simulink model "model"  (R2018a)
settings: Solver=VariableStepAuto  StartTime=0.0  StopTime=0.01  MaxStep=1e-5  RelTol=1e-3
values from neighbouring files (symbols this model uses):
  Cp = 1/(4*pi^2*f^2*Lp)    (= 1.42505180932e-08)    [parametric_simulation.m]
  Cs = 1/(4*pi^2*f^2*Ls)    (= 1.63158105704e-08)    [parametric_simulation.m]
  fop = 156    [parametric_simulation.m]
  R_Load = 10    [parametric_simulation.m]
  Vin_peak = 127    [parametric_simulation.m]
libraries: powerlib x42
settings Model: Creator=user  LastModifiedBy=enes_

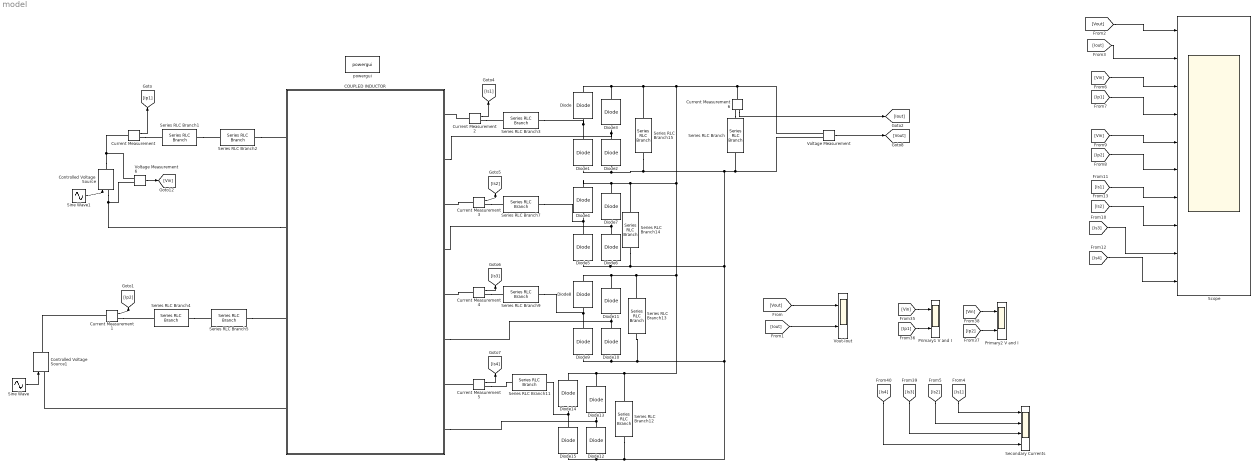
== system model ==
  COUPLED INDUCTOR : Subsystem
  Controlled Voltage Source : powerlib/Electrical Sources/Controlled Voltage Source  Initialize=on  Source_Type=AC  Amplitude=0  Phase=0  Frequency=0  Measurements=None
  Controlled Voltage Source1 : powerlib/Electrical Sources/Controlled Voltage Source  Initialize=on  Source_Type=AC  Amplitude=0  Phase=0  Frequency=0  Measurements=None
  Current Measurement{,1..6} (7 alike) : powerlib/Measurements/Current Measurement  PhasorSimulation=off  OutputType=Complex  PSBequivalent=0
  Diode{,1..15} (16 alike) : powerlib/Power Electronics/Diode  Ron=0.001  Lon=0  Vf=0.8  IC=0  UseSnubber=0  Rs=inf  Cs=250e-9  Measurements=off
  Primary1 V and I : Scope  NumInputPorts=2
  Primary2 V and I : Scope  NumInputPorts=2
  Scope : Scope  NumInputPorts=10
  Secondary Currents : Scope  NumInputPorts=4
  Series RLC Branch : powerlib/Elements/Series RLC Branch  LConnTagsString=__new0  RConnTagsString=__new0  BranchType=R  Resistance=R_Load  Inductance=1e-3  SetiL0=off  InitialCurrent=0  Capacitance=1e-6  Setx0=off  InitialVoltage=0  Measurements=None
  Series RLC Branch1 : powerlib/Elements/Series RLC Branch  LConnTagsString=__new0  RConnTagsString=__new0  BranchType=R  Resistance=0.01  Inductance=1e-3  SetiL0=off  InitialCurrent=0  Capacitance=1e-6  Setx0=off  InitialVoltage=0  Measurements=None
  Series RLC Branch{3,7,9,11} (4 alike) : powerlib/Elements/Series RLC Branch  LConnTagsString=__new0  RConnTagsString=__new0  BranchType=C  Resistance=0.01  Inductance=1e-3  SetiL0=off  InitialCurrent=0  Capacitance=Cs  Setx0=off  InitialVoltage=0  Measurements=None
  Series RLC Branch{12..15} (4 alike) : powerlib/Elements/Series RLC Branch  LConnTagsString=__new0  RConnTagsString=__new0  BranchType=C  Resistance=70  Inductance=1e-3  SetiL0=off  InitialCurrent=0  Capacitance=1e-6  Setx0=off  InitialVoltage=0  Measurements=None
  Series RLC Branch2 : powerlib/Elements/Series RLC Branch  LConnTagsString=__new0  RConnTagsString=__new0  BranchType=C  Resistance=0.01  Inductance=1e-3  SetiL0=off  InitialCurrent=0  Capacitance=Cp  Setx0=off  InitialVoltage=0  Measurements=None
  Series RLC Branch4 : powerlib/Elements/Series RLC Branch  LConnTagsString=__new0  RConnTagsString=__new0  BranchType=R  Resistance=0.01  Inductance=1e-3  SetiL0=off  InitialCurrent=0  Capacitance=1e-6  Setx0=off  InitialVoltage=0  Measurements=None
  Series RLC Branch5 : powerlib/Elements/Series RLC Branch  LConnTagsString=__new0  RConnTagsString=__new0  BranchType=C  Resistance=0.01  Inductance=1e-3  SetiL0=off  InitialCurrent=0  Capacitance=Cp  Setx0=off  InitialVoltage=0  Measurements=None
  Sine Wave : Sin  Amplitude=Vin_peak  Frequency=fop*1000*2*pi  SampleTime=0
  Sine Wave1 : Sin  Amplitude=Vin_peak  Frequency=fop*1000*2*pi  SampleTime=0
  Voltage Measurement : powerlib/Measurements/Voltage Measurement  PhasorSimulation=off  OutputType=Complex  PSBequivalent=0
  Voltage Measurement6 : powerlib/Measurements/Voltage Measurement  PhasorSimulation=off  OutputType=Complex  PSBequivalent=0
  Vout-Iout : Scope  NumInputPorts=2
  powergui : powerlib/powergui  Priority=1  SimulationMode=Continuous  SampleTime=50e-6  frequency=60  Iterations=50  frequencyindice=0  Pbase=100e6  ErrMax=1e-4  UnitsV=kV  UnitsW=MW  buscounter=0  FunctionMessages=off  echomessages=off  EnableUseOfTLC=off  CurrentSourceSwitches=off  DisableSnubberDevices=off  DisableRonSwitches=off  DisableVfSwitches=off  DisplayEquations=off  SolverType=Tustin/Backward Euler (TBE)  Interpol=off  ExternalGateDelay=off  methode=off  Ts=100  x0status=blocks  SPID=on  SwTol=0  HookPort=off  RestoreLinks=warning  ResistiveCurrentMeasurement=off  Frange=[0:2:500]  Ylog=off  Xlog=on  ShowGrid=off  save=off  variable=ZData  structure=0  ZoomFFT=off  StartTime=0.0  cycles=1  DisplayStyle=1  fundamental=60  FreqAxis=off  MaxFrequency=1000  frequencyindicesteady=1  RmsSteady=1  display=off
  wires:
  [Ip1] -> Primary1 V and I/2
  [Vin] -> Primary1 V and I/1
  [Vin] -> Primary2 V and I/1
  Current Measurement/1 -> [Ip1]
  Current Measurement4/1 -> [Is3]
  Current Measurement1/1 -> [Ip2]
  [Vout] -> Vout-Iout/1
  Sine Wave1/1 -> Controlled Voltage Source/1
  Current Measurement3/1 -> [Is2]
  Voltage Measurement/1 -> [Vout]
  Sine Wave/1 -> Controlled Voltage Source1/1
  [Ip2] -> Primary2 V and I/2
  Current Measurement2/1 -> [Is1]
  Current Measurement5/1 -> [Is4]
  Voltage Measurement6/1 -> [Vin]
  [Is1] -> Secondary Currents/1
  [Is2] -> Secondary Currents/2
  [Is3] -> Secondary Currents/3
  [Is4] -> Secondary Currents/4
  Current Measurement6/1 -> [Iout]
  [Iout] -> Vout-Iout/2
  [Iout] -> Scope/2
  [Vout] -> Scope/1
  [Vin] -> Scope/3
  [Ip1] -> Scope/4
  [Vin] -> Scope/5
  [Ip2] -> Scope/6
  [Is1] -> Scope/7
  [Is2] -> Scope/8
  [Is3] -> Scope/9
  [Is4] -> Scope/10
  connections:
  Series RLC Branch1/LConn1 -- Series RLC Branch2/LConn1
  Series RLC Branch4/LConn1 -- Series RLC Branch5/LConn1
  Controlled Voltage Source/RConn1 -- Current Measurement/LConn1 -- Voltage Measurement6/LConn1
  Series RLC Branch5/RConn1 -- COUPLED INDUCTOR/RConn3
  Series RLC Branch2/RConn1 -- COUPLED INDUCTOR/RConn1
  COUPLED INDUCTOR/RConn2 -- Controlled Voltage Source/LConn1 -- Voltage Measurement6/LConn2
  Current Measurement1/LConn1 -- Controlled Voltage Source1/RConn1
  Current Measurement/RConn1 -- Series RLC Branch1/RConn1
  Current Measurement3/RConn1 -- Series RLC Branch7/LConn1
  Current Measurement4/LConn1 -- COUPLED INDUCTOR/LConn5
  Current Measurement5/RConn1 -- Series RLC Branch11/LConn1
  Current Measurement2/LConn1 -- COUPLED INDUCTOR/LConn1
  Current Measurement5/LConn1 -- COUPLED INDUCTOR/LConn7
  Current Measurement2/RConn1 -- Series RLC Branch3/LConn1
  COUPLED INDUCTOR/RConn4 -- Controlled Voltage Source1/LConn1
  Current Measurement3/LConn1 -- COUPLED INDUCTOR/LConn3
  Current Measurement4/RConn1 -- Series RLC Branch9/LConn1
  Current Measurement1/RConn1 -- Series RLC Branch4/RConn1
  Diode1/RConn1 -- Series RLC Branch3/RConn1 -- Diode/LConn1
  Diode3/LConn1 -- COUPLED INDUCTOR/LConn2 -- Diode2/RConn1
  Diode14/RConn1 -- Current Measurement6/LConn1 -- Voltage Measurement/LConn1 -- Diode3/RConn1 -- Diode/RConn1 -- Series RLC Branch15/LConn1 -- Diode4/RConn1 -- Diode7/RConn1 -- Series RLC Branch14/LConn1 -- Diode8/RConn1 -- Diode11/RConn1 -- Series RLC Branch13/LConn1 -- Series RLC Branch12/LConn1 -- Diode13/RConn1
  Series RLC Branch12/RConn1 -- Voltage Measurement/LConn2 -- Series RLC Branch/RConn1 -- Diode2/LConn1 -- Diode1/LConn1 -- Series RLC Branch15/RConn1 -- Series RLC Branch14/RConn1 -- Diode6/LConn1 -- Diode5/LConn1 -- Series RLC Branch13/RConn1 -- Diode9/LConn1 -- Diode10/LConn1 -- Diode12/LConn1 -- Diode15/LConn1
  Diode7/LConn1 -- COUPLED INDUCTOR/LConn4 -- Diode6/RConn1
  Diode5/RConn1 -- Series RLC Branch7/RConn1 -- Diode4/LConn1
  Diode9/RConn1 -- Series RLC Branch9/RConn1 -- Diode8/LConn1
  Diode11/LConn1 -- COUPLED INDUCTOR/LConn6 -- Diode10/RConn1
  Diode13/LConn1 -- COUPLED INDUCTOR/LConn8 -- Diode12/RConn1
  Diode15/RConn1 -- Series RLC Branch11/RConn1 -- Diode14/LConn1
  Current Measurement6/RConn1 -- Series RLC Branch/LConn1

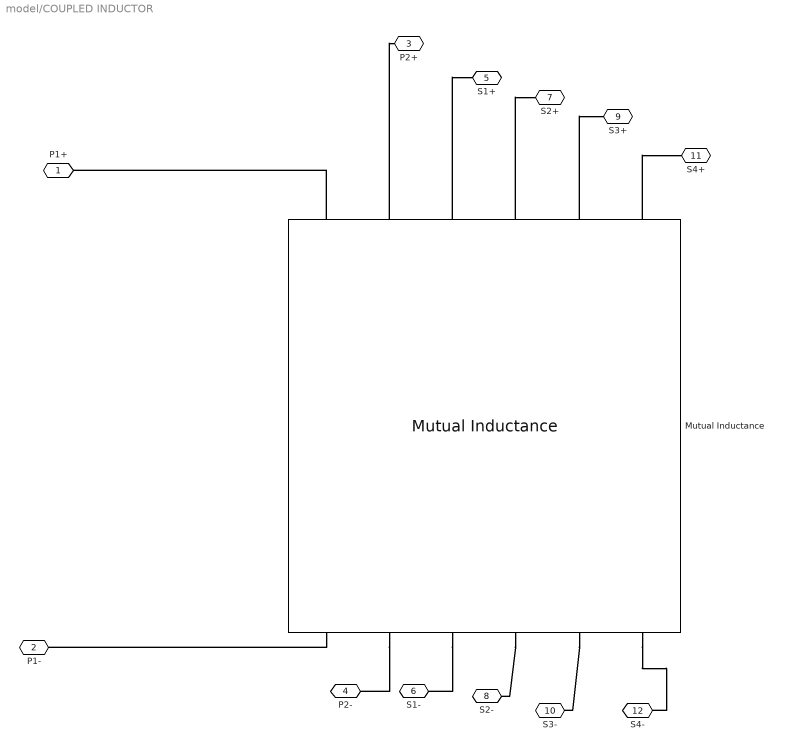
== system model/COUPLED INDUCTOR ==
  Mutual Inductance : powerlib/Elements/Mutual Inductance  LConnTagsString=a|b|c|L4|L5|L6  RConnTagsString=A|B|C|R4|R5|R6  TypeOfMutual=Generalized mutual inductance  NumberOfWindings=6  SelfImpedance1=[1.1 1.1e-03]  SelfImpedance2=[ 1.1 1.1e-03]  ThreeWindings=on  SelfImpedance3=[ 1.1 1.1e-03]  MutualImpedance=[1.0 1.0e-03]  InductanceMatrix=L  ResistanceMatrix=R  Measurements=None
      settings: AttributesFormatString=\n  SourceProductName=Simscape Power Systems  SourceProductBaseCode=PS
  P1+ : PMIOPort  Side=Right
  P1- : PMIOPort  Port=2  Side=Right
  P2+ : PMIOPort  Port=3  Side=Right
  P2- : PMIOPort  Port=4  Side=Right
  S1+ : PMIOPort  Port=5  Side=Left
  S1- : PMIOPort  Port=6  Side=Left
  S2+ : PMIOPort  Port=7  Side=Left
  S2- : PMIOPort  Port=8  Side=Left
  S3+ : PMIOPort  Port=9  Side=Left
  S3- : PMIOPort  Port=10  Side=Left
  S4+ : PMIOPort  Port=11  Side=Left
  S4- : PMIOPort  Port=12  Side=Left
  connections:
  Mutual Inductance/LConn2 -- P2-/RConn1
  Mutual Inductance/LConn5 -- S3-/RConn1
  Mutual Inductance/RConn5 -- S3+/RConn1
  Mutual Inductance/RConn4 -- S2+/RConn1
  Mutual Inductance/LConn6 -- S4-/RConn1
  Mutual Inductance/RConn1 -- P1+/RConn1
  Mutual Inductance/LConn1 -- P1-/RConn1
  Mutual Inductance/RConn2 -- P2+/RConn1
  Mutual Inductance/LConn4 -- S2-/RConn1
  Mutual Inductance/LConn3 -- S1-/RConn1
  Mutual Inductance/RConn3 -- S1+/RConn1
  Mutual Inductance/RConn6 -- S4+/RConn1
